simulink model "Practica_6_slx"  (R2023a)
settings: Solver=VariableStepAuto  StartTime=0.0  StopTime=0.003  MaxStep=0.0000001  RelTol=1e-3
values from neighbouring files (symbols this model uses):
  C1 = 1e-7    (= 1e-07)    [Practica_6_f.m]    (also in Practica_6_slx_code.m)
  C2 = C1    (= 1e-07)    [Practica_6_f.m]    (also in Practica_6_slx_code.m)
  R1 = 1000    [Practica_6_f.m]    (also in Practica_6_slx_code.m)
  R2 = R1    (= 1000)    [Practica_6_f.m]    (also in Practica_6_slx_code.m)
  R3 = 10000    [Practica_6_f.m]    (also in Practica_6_slx_code.m)
  R4 = 15000    [Practica_6_f.m]    (also in Practica_6_slx_code.m)
  V7 = 1    [Practica_6_f.m]    (also in Practica_6_slx_code.m)
libraries: fl_lib x12, nesl_utility x3
settings Model: Creator=Peri_XP  LastModifiedBy=mluser

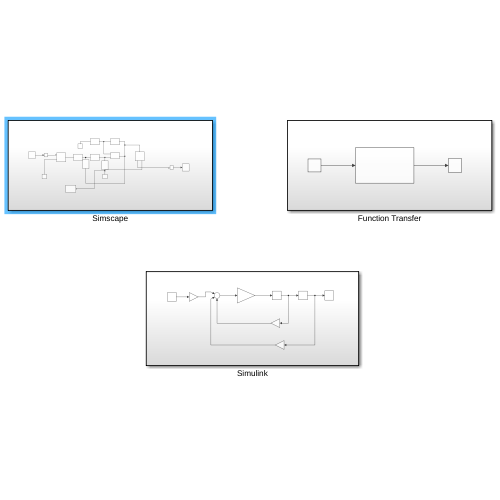
[thumbnail: Simulink's stored preview of the top-level diagram]
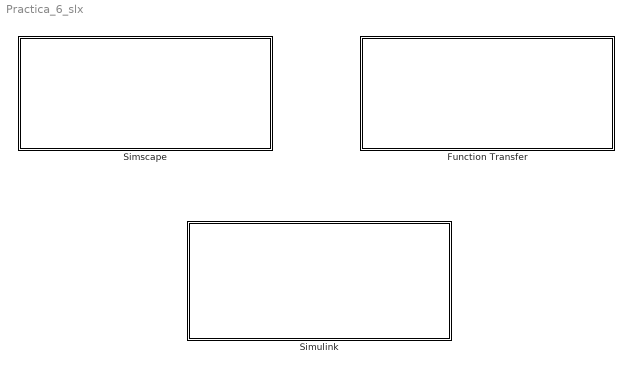
== system Practica_6_slx ==
  Function Transfer : Subsystem
  Simscape : Subsystem
  Simulink : Subsystem

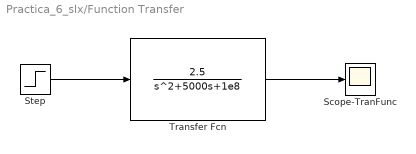
== system Practica_6_slx/Function Transfer ==
  Scope-TranFunc : Scope
  Step : Step  Time=0  After=V7  SampleTime=0
  Transfer Fcn : TransferFcn  Numerator=[2.5]  Denominator=[1 5000 1e8]
  wires:
  Step/1 -> Transfer Fcn/1
  Transfer Fcn/1 -> Scope-TranFunc/1

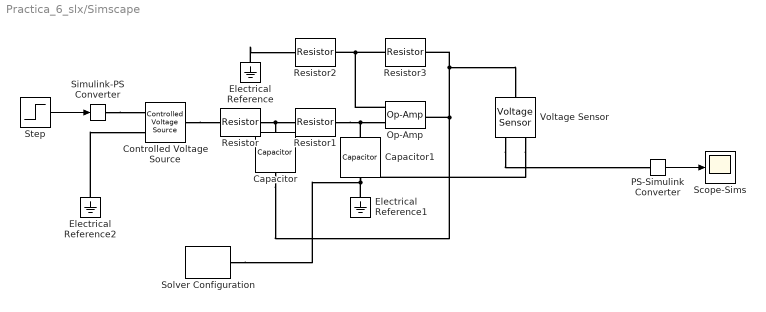
== system Practica_6_slx/Simscape ==
  Capacitor : fl_lib/Electrical/Electrical Elements/Capacitor  c=C1 F  r=1e-6 Ohm  g=0 1/Ohm  i_specify=off  i_priority=None  i=0 A  i_nominal_specify=off  i_nominal_unit=A  i_nominal_value=1  v_specify=off  v_priority=None  v=0 V  v_nominal_specify=off  v_nominal_unit=V  v_nominal_value=1  vc_specify=off  vc_priority=High  vc=0 V  vc_nominal_specify=off  vc_nominal_unit=V  vc_nominal_value=1
  Capacitor1 : fl_lib/Electrical/Electrical Elements/Capacitor  c=C2 F  r=1e-6 Ohm  g=0 1/Ohm  i_specify=off  i_priority=None  i=0 A  i_nominal_specify=off  i_nominal_unit=A  i_nominal_value=1  v_specify=off  v_priority=None  v=0 V  v_nominal_specify=off  v_nominal_unit=V  v_nominal_value=1  vc_specify=off  vc_priority=High  vc=0 V  vc_nominal_specify=off  vc_nominal_unit=V  vc_nominal_value=1
  Controlled Voltage Source : fl_lib/Electrical/Electrical Sources/Controlled Voltage Source
  Electrical Reference : fl_lib/Electrical/Electrical Elements/Electrical Reference
  Electrical Reference1 : fl_lib/Electrical/Electrical Elements/Electrical Reference
  Electrical Reference2 : fl_lib/Electrical/Electrical Elements/Electrical Reference
  Op-Amp : fl_lib/Electrical/Electrical Elements/Op-Amp  outI_specify=off  outI_priority=None  outI=0 A  outI_nominal_specify=off  outI_nominal_unit=A  outI_nominal_value=1
  PS-Simulink Converter : nesl_utility/PS-Simulink Converter  PhysicalDomain=network_engine_domain  SubClassName=ps_output  LeftPortType=input  RightPortType=output  PseudoPeriodic=off  Frequencies=[]  VectorFormat=inherit  Unit=inherit  AffineConversion=off
  Resistor : fl_lib/Electrical/Electrical Elements/Resistor  R=R1 Ohm  i_specify=off  i_priority=None  i=0 A  i_nominal_specify=off  i_nominal_unit=A  i_nominal_value=1  v_specify=off  v_priority=None  v=0 V  v_nominal_specify=off  v_nominal_unit=V  v_nominal_value=1
  Resistor1 : fl_lib/Electrical/Electrical Elements/Resistor  R=R2 Ohm  i_specify=off  i_priority=None  i=0 A  i_nominal_specify=off  i_nominal_unit=A  i_nominal_value=1  v_specify=off  v_priority=None  v=0 V  v_nominal_specify=off  v_nominal_unit=V  v_nominal_value=1
  Resistor2 : fl_lib/Electrical/Electrical Elements/Resistor  R=R3 Ohm  i_specify=off  i_priority=None  i=0 A  i_nominal_specify=off  i_nominal_unit=A  i_nominal_value=1  v_specify=off  v_priority=None  v=0 V  v_nominal_specify=off  v_nominal_unit=V  v_nominal_value=1
  Resistor3 : fl_lib/Electrical/Electrical Elements/Resistor  R=R4 Ohm  i_specify=off  i_priority=None  i=0 A  i_nominal_specify=off  i_nominal_unit=A  i_nominal_value=1  v_specify=off  v_priority=None  v=0 V  v_nominal_specify=off  v_nominal_unit=V  v_nominal_value=1
  Scope-Sims : Scope
  Simulink-PS Converter : nesl_utility/Simulink-PS Converter  PhysicalDomain=network_engine_domain  SubClassName=ps_input  LeftPortType=input  RightPortType=output  PseudoPeriodic=off  Frequencies=[]  NoiseDistribution=none  NoiseParameters=[]  Unit=1  AffineConversion=off  FilteringAndDerivatives=provide  SimscapeFilterOrder=1  InputFilterTimeConstant=0.001  UdotUserProvided=0
  Solver Configuration : nesl_utility/Solver Configuration  PhysicalDomain=network_engine_domain  SubClassName=solver  LeftPortType=input  RightPortType=generic  Tones=[]  Harmonics=[]  SimulateNoise=off  Profile=off  UseLocalSampling=off  EnableSwitchedLinearOptims=on  FrequencyDomain=off  UseCCode=off  RelTol=0.001  AbsTol=0.001  MinStep=1e-09  ToWorkspace=off  RevertToSquareIcSolve=off  NumHomotopyIterations=100  PhasorMode=off  PhasorModeNumHarmonics=1  ConsistencySolver=NEWTON_XTOL_AFTER_FTOL  IndexReductionMethod=DerivativeReplacement  DoDC=off  ResidualTolerance=1e-09  ConsistencyTolSource=GLOBAL  ConsistencyAbsTol=0.001  ConsistencyRelTol=0.001  ConsistencyTolFactor=0.001  UseLocalSolver=off  LocalSolverChoice=NE_BACKWARD_EULER_ADVANCER  ResolveIndetEquations=on  FunctionEvalNumThread=1  LocalSolverSampleTime=0.001  DoFixedCost=off  MaxNonlinIter=3  MaxModeIter=2  ComputeImpulses=off  ImpulseIterations=2  LinearAlgebra=auto  LinearAlgebraNumThread=0  EquationFormulation=NE_TIME_EF  DelaysMemoryBudget=1024  AutomaticFiltering=on  FilteringTimeConstant=0.001  PartitionStorageMethod=AS_NEEDED  PartitionMemoryBudget=1024  PartitionMethod=ROBUST
  Step : Step  Time=0  SampleTime=0
  Voltage Sensor : fl_lib/Electrical/Electrical Sensors/Voltage Sensor
  wires:
  Step/1 -> Simulink-PS Converter/1
  PS-Simulink Converter/1 -> Scope-Sims/1
  connections:
  Resistor/RConn1 -- Capacitor/LConn1 -- Resistor1/LConn1
  Capacitor/RConn1 -- Voltage Sensor/LConn1 -- Resistor3/RConn1 -- Op-Amp/RConn1
  Resistor3/LConn1 -- Op-Amp/LConn2 -- Resistor2/RConn1
  Voltage Sensor/RConn1 -- PS-Simulink Converter/LConn1
  Resistor1/RConn1 -- Capacitor1/LConn1 -- Op-Amp/LConn1
  Electrical Reference1/LConn1 -- Capacitor1/RConn1 -- Voltage Sensor/RConn2 -- Solver Configuration/RConn1
  Electrical Reference/LConn1 -- Resistor2/LConn1
  Electrical Reference2/LConn1 -- Controlled Voltage Source/RConn2
  Controlled Voltage Source/LConn1 -- Resistor/LConn1
  Simulink-PS Converter/RConn1 -- Controlled Voltage Source/RConn1

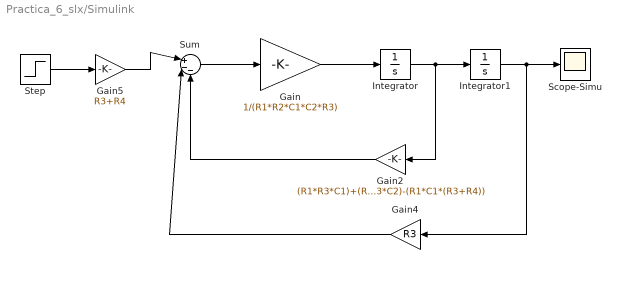
== system Practica_6_slx/Simulink ==
  Gain : Gain  Gain=1/(R1*R2*C1*C2*R3)
  Gain2 : Gain  Gain=(R1*R3*C1)+(R2*R3*C2)+(R1*R3*C2)-(R1*C1*(R3+R4))
  Gain4 : Gain  Gain=R3
  Gain5 : Gain  Gain=R3+R4
  Integrator : Integrator
  Integrator1 : Integrator
  Scope-Simu : Scope
  Step : Step  Time=0  After=V7  SampleTime=0
  Sum : Sum  Inputs=|+--
  wires:
  Sum/1 -> Gain/1
  Gain5/1 -> Sum/1
  Gain2/1 -> Sum/3
  Gain4/1 -> Sum/2
  Integrator1/1 -> Gain4/1, Scope-Simu/1
  Step/1 -> Gain5/1
  Integrator/1 -> Gain2/1, Integrator1/1
  Gain/1 -> Integrator/1
